simulink subsystem "gfmWind"  (R2025a)
settings: Solver=VariableStepAuto  StartTime=0.0  StopTime=10.0  RelTol=1e-3
model mask{Control=VSM Using DC Link Voltage, V_ref=V_ref, Q_ref=Q_ref, Kq=Kq_dc, Kt=Kt, KqI=Kq, Kp=Kp, Kd=Kd, Kj=Kj, H=H, D=D, Vd_ref=0, frequency1=0, frequency=0, Spref=Curtailed Power Operation, tstart=0, Vslope=0, Pstart=0, Pslope=0, x_vir=0, x_vir1=0, r_vir1=0, Imax1=0, Imax=0, r_vir=0, Kpq_mpp=Lq*alpha, Kpd_mpp=Ld*alpha, Kiq_mpp=Rs*alpha, Kid_mpp=Rs*alpha, Kpq=Lq*alpha, Kpd=Ld*alpha, Kiq=Rs*alpha, Kid=Rs*alpha, Kp_dc_sm=Kp_dc_sm, Ki_dc_sm=Ki_dc_sm, wt1=0, rt1=0, pitch1=0, cp1=0, airDensity1=0, TSR1=0, Radius1=0, wt=0.01, rt=0.01, pitch=pitch, cp=cp, airDensity=airDensity, Radius=turbineRadius, TSR=TSR, Inertia1=0, Inertia=0, psim1=0, p1=0, Rs1=0, Lq1=0, Ld1=0, Ld=Ld, Lq=Lq, Rs=Rs, p=p, psim=psim}
  mask prompts: Control "GFM Controller"; V_ref "Voltage Reference (PU)"; Q_ref "Reactive Power Reference"; Kq "Reactive Power Droop"; Kt "Tracking Coefficient"; KqI "VSM Reactive power droop"; Kp "VSM frequency droop"; Kd "Damping Coefficient"; Kj "Inertia Coefficient"; H "VSM Inertia"; D "VSM damping"; Vd_ref "Volatge Reference d-axis"; frequency1 "Frequency reference"; frequency "Reference frequency"; Spref "Select Real Power Rference (MW)"; tstart "Start time of Voltage ramp (s)"; Vslope "Slope of Voltage ramp (pu)"; Pstart "Start time of Power ramp (s)"; Pslope "Slope of Power ramp (pu)"; x_vir "Virtual reactance"; x_vir1 "Virtual reactance"; r_vir1 "Virtual resistance"; Imax1 "Current limit"; Imax "Current limit"; r_vir "Virtual resistance"; Kpq_mpp "Q-axis Proportional Gain"; Kpd_mpp "D-axis Proportional Gain"; Kiq_mpp "Q-axis Integral Gain"; Kid_mpp "D-axis Integral Gain"; Kpq "q-axis proportional Gain"; Kpd "D-axis proportional Gain"; Kiq "q-axis integral Gain"; Kid "D-axis integral Gain"; Kp_dc_sm "Prportional Gain of Dc-link Controller"; Ki_dc_sm "Integral Gain of DC-link Controller"; wt1 "Wind Velocity Threshold"; rt1 "Rotational Velocity Threshold"; pitch1 "Pitch Angle Vector"; cp1 "Power Coefficient Table"; airDensity1 "Air Density"; TSR1 "Tip Speed Ratio"; Radius1 "Radius of Turbine"; wt "Wind Velocity Threshold"; rt "Rotational Velocity Threshold"; pitch "Turbine Pitch Angle Vector"; cp "Power Coefficient"; airDensity "Air Density"; Radius "Turbine Radius"; TSR "Tip Speed Ratio"; Inertia1 "Turbine Inertia"; Inertia "Turbine Inertia"; psim1 "PM Flux Linkage"; p1 "Number of Pole Pairs"; Rs1 "Stator Resistance (Ohms)"; Lq1 "Stator Q-axis inductance (H)"; Ld1 "Stator D-axis inductance (H)"; Ld "Stator D-axis inductance (H)"; Lq "Stator Q-axis inductance (H)"; Rs "Stator Resistance (Ohms)"; p "Number of Pole Pairs"; psim "PMSM Flux linkage (Wb)"
settings Model: Creator=rajarshd  LastModifiedBy=rajarshd
settings RTWCC: GPUComputeCapability=3.5

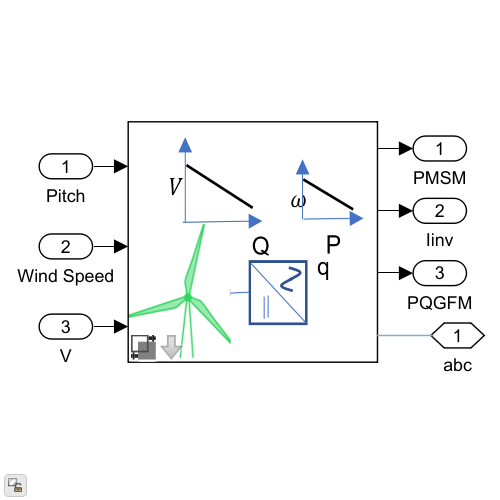
[thumbnail: Simulink's stored preview of the top-level diagram]
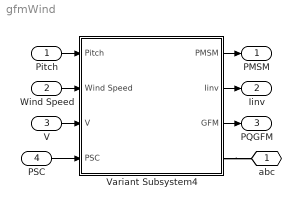
== system gfmWind ==
  Pitch : Inport
  Wind Speed : Inport  Port=2
  V : Inport  Port=3
  PSC : Inport  Port=4
  Variant Subsystem4 : Subsystem  Variant=on  VariantControlMode=label  LabelModeActiveChoice=WindVSMControlDClink  PropagateVariantConditions=on  mask{Control=VSM Using DC Link Voltage, KqI=KqI, Q_ref=Q_ref, Kp=Kp, H=H, D=D, V_ref=V_ref, Kq=Kq, Kt=Kt, Kj=Kj, Kd=Kd, Vd_ref=Vd_ref, frequency=frequency, frequency1=frequency1, Spref=Curtailed Power Operation, Pslope=Pslope, Pstart=Pstart, Vslope=Vslope, tstart=tstart, x_vir1=x_vir1, x_vir=x_vir, r_vir=r_vir, r_vir1=r_vir1, Imax=Imax, Imax1=Imax1, Kid=Kid, Kiq=Kiq, Kpd=Kpd, Kpq=Kpq, Ki_dc_sm=Ki_dc_sm, Kp_dc_sm=Kp_dc_sm, Kpq_mpp=Kpq_mpp, Kpd_mpp=Kpd_mpp, Kid_mpp=Kid_mpp, Kiq_mpp=Kiq_mpp, psim1=psim1, p1=p1, Rs1=Rs1, Lq1=Lq1, Ld1=Ld1, Ld=Ld, Lq=Lq, p=p, psim=psim, Rs=Rs, wt1=wt1, rt1=rt1, pitch1=pitch1, cp1=cp1, TSR1=TSR1, Radius1=Radius1, airDensity1=airDensity1, Radius=Radius, TSR=TSR, airDensity=airDensity, cp=cp, pitch=pitch, rt=rt, wt=wt, Inertia1=Inertia1, Inertia=Inertia}
      mask prompts: Control "GFM Controller"; KqI "VSM Reactive power droop"; Q_ref "Reactive Power Reference"; Kp "VSM frequency droop"; H "VSM Inertia"; D "VSM damping"; V_ref "Voltage Reference (PU)"; Kq "Reactive Power Droop"; Kt "Tracking Cofficient"; Kj "Inertia Cofficient"; Kd "Damping Cofficient"; Vd_ref "Volatge Reference d-axis"; frequency "Reference frequency"; frequency1 "Frequency reference"; Spref "Select Real Power Rference (MW)"; Pslope "Slope of Power ramp (pu)"; Pstart "Start time of Power ramp (s)"; Vslope "Slope of Voltage ramp (pu)"; tstart "Start time of Voltage ramp (s)"; x_vir1 "Virtual reactance"; x_vir "Virtual reactance"; r_vir "Virtual resistance"; r_vir1 "Virtual resistance"; Imax "Current limit"; Imax1 "Current limit"; Kid "D-axis integral Gain"; Kiq "q-axis integral Gain"; Kpd "D-axis proportional Gain"; Kpq "q-axis proportional Gain"; Ki_dc_sm "Integral Gain of DC-link Controller"; Kp_dc_sm "Prportional Gain of Dc-link Controller"; Kpq_mpp "Q-axis Proportional Gain"; Kpd_mpp "D-axis Proportional Gain"; Kid_mpp "D-axis Integral Gain"; Kiq_mpp "Q-axis Integral Gain"; psim1 "PM Flux Linkage"; p1 "Number of Pole Pairs"; Rs1 "Stator Resistance (Ohms)"; Lq1 "Stator Q-axis inductance (H)"; Ld1 "Stator D-axis inductance (H)"; Ld "Stator D-axis inductance (H)"; Lq "Stator Q-axis inductance (H)"; p "Number of Pole Pairs"; psim "PMSM Flux linkage (Wb)"; Rs "Stator Resistance (Ohms)"; wt1 "Wind Velocity Threshold"; rt1 "Rotational Velocity Threshold"; pitch1 "Pitch Angle Vector"; cp1 "Power Cofficient Table"; TSR1 "Tip Speed Ratio"; Radius1 "Radious of Turbine"; airDensity1 "Air Density"; Radius "Turbine Radious"; TSR "Tip Speed Ratio"; airDensity "Air Density"; cp "Power Cofficient"; pitch "Turbine Pitch Angle Vector"; rt "Rotational Velocity Threshold"; wt "Wind Velocity Threshold"; Inertia1 "Turbine Inertia"; Inertia "Turbine Inertia"
      mask init:
      | Choice = get_param(gcb,'Control');
      | switch Choice
      |     case 'VSM Using DC Link Voltage'
      |         set_param(gcb, 'LabelModeActiveChoice', 'WindVSMControlDClink')
      |     case 'VSM Using Turbine Inertia'
      |          set_param(gcb, 'LabelModeActiveChoice', 'WindVSMControlTurbineInertia')
      |    otherwise
      |         disp('Choose proper active power control method')
      | end
      mask TypeOptions Control: VSM Using Turbine Inertia | VSM Using DC Link Voltage
      mask Callback Control:
      | h = Simulink.Mask.get(gcb);
      | Choice = get_param(gcb,'Control');
      | switch Choice
      |     case 'VSM Using DC Link Voltage'
      |         set_param(gcb, 'LabelModeActiveChoice', 'WindVSMControlDClink')
      |     case 'VSM Using Turbine Inertia'
      |          set_param(gcb, 'LabelModeActiveChoice', 'WindVSMControlTurbineInertia')
      | end
      mask TypeOptions KqI: VSM Inertia/KqI
      mask TypeOptions Q_ref: VSM DC/Q_ref
      mask TypeOptions Kp: VSM Inertia/Kp
      mask TypeOptions H: VSM Inertia/H
      mask TypeOptions D: VSM Inertia/D
      mask TypeOptions V_ref: VSM DC/V_ref
      mask TypeOptions Kq: VSM DC/Kq
      mask TypeOptions Kt: VSM DC/Kt
      mask TypeOptions Kj: VSM DC/Kj
      mask TypeOptions Kd: VSM DC/Kd
      mask TypeOptions Vd_ref: VSM Inertia/Vd_ref
      mask TypeOptions frequency: VSM Inertia/frequency
      mask TypeOptions frequency1: VSM DC/frequency1
      mask TypeOptions Spref: VSM Inertia/Spref
      mask TypeOptions Pslope: VSM Inertia/Pslope
      mask TypeOptions Pstart: VSM Inertia/Pstart
      mask TypeOptions Vslope: VSM Inertia/Vslope
      mask TypeOptions tstart: VSM Inertia/tstart
      mask TypeOptions x_vir1: VSM DC/x_vir1
      mask TypeOptions x_vir: VSM Inertia/x_vir
      mask TypeOptions r_vir: VSM Inertia/r_vir
      mask TypeOptions r_vir1: VSM DC/r_vir1
      mask TypeOptions Imax: VSM Inertia/Imax
      mask TypeOptions Imax1: VSM DC/Imax1
      mask TypeOptions Kid: VSM Inertia/Kid
      mask TypeOptions Kiq: VSM Inertia/Kiq
      mask TypeOptions Kpd: VSM Inertia/Kpd
      mask TypeOptions Kpq: VSM Inertia/Kpq
      mask TypeOptions Ki_dc_sm: VSM Inertia/Ki_dc_sm
      mask TypeOptions Kp_dc_sm: VSM Inertia/Kp_dc_sm
      mask TypeOptions Kpq_mpp: VSM DC/Kpq_mpp
      mask TypeOptions Kpd_mpp: VSM DC/Kpd_mpp
      mask TypeOptions Kid_mpp: VSM DC/Kid_mpp
      mask TypeOptions Kiq_mpp: VSM DC/Kiq_mpp
      mask TypeOptions psim1: VSM Inertia/psim1
      mask TypeOptions p1: VSM Inertia/p1
      mask TypeOptions Rs1: VSM Inertia/Rs1
      mask TypeOptions Lq1: VSM Inertia/Lq1
      mask TypeOptions Ld1: VSM Inertia/Ld1
      mask TypeOptions Ld: VSM DC/Ld
      mask TypeOptions Lq: VSM DC/Lq
      mask TypeOptions p: VSM DC/p
      mask TypeOptions psim: VSM DC/psim
      mask TypeOptions Rs: VSM DC/Rs
      mask TypeOptions wt1: VSM Inertia/wt1
      mask TypeOptions rt1: VSM Inertia/rt1
      mask TypeOptions pitch1: VSM Inertia/pitch1
      mask TypeOptions cp1: VSM Inertia/cp1
      mask TypeOptions TSR1: VSM Inertia/TSR1
      mask TypeOptions Radius1: VSM Inertia/Radius1
      mask TypeOptions airDensity1: VSM Inertia/airDensity1
      mask TypeOptions Radius: VSM DC/Radius
      mask TypeOptions TSR: VSM DC/TSR
      mask TypeOptions airDensity: VSM DC/airDensity
      mask TypeOptions cp: VSM DC/cp
      mask TypeOptions pitch: VSM DC/pitch
      mask TypeOptions rt: VSM DC/rt
      mask TypeOptions wt: VSM DC/wt
      mask TypeOptions Inertia1: VSM Inertia/Inertia1
      mask TypeOptions Inertia: VSM DC/Inertia
      mask DialogControl Container4 Prompt: VSM Parameters
      mask DialogControl Container8 Prompt: Fault Ridethrough Parameters
      mask DialogControl Container5 Prompt: PMSM Controller
      mask DialogControl Container6 Prompt: PMSM Parameters
      mask DialogControl Container7 Prompt: Wind Turbine Parameters
      mask Display: image('WindGFM.png')
  abc : PMIOPort  Side=Right
  PMSM : Outport
  Iinv : Outport  Port=2
  PQGFM : Outport  Port=3
  wires:
  Variant Subsystem4/3(GFM) -> PQGFM/1
  Wind Speed/1 -> Variant Subsystem4/2(Wind Speed)
  V/1 -> Variant Subsystem4/3(V)
  Variant Subsystem4/1(PMSM) -> PMSM/1
  Pitch/1 -> Variant Subsystem4/1(Pitch)
  Variant Subsystem4/2(Iinv) -> Iinv/1
  PSC/1 -> Variant Subsystem4/4(PSC)
  connections:
  Variant Subsystem4/RConn1 -- abc/RConn1

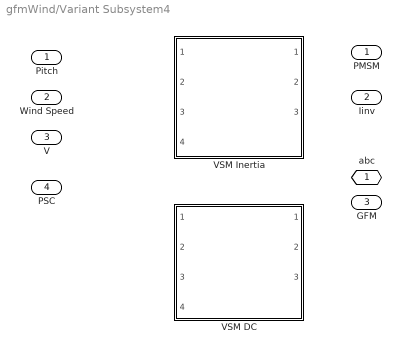
== system gfmWind/Variant Subsystem4 ==
  Pitch : Inport
  Wind Speed : Inport  Port=2
  V : Inport  Port=3
  PSC : Inport  Port=4
  VSM DC : Subsystem  VariantControl=WindVSMControlDClink  ReferencedSubsystem=WindGFMCap  x_vir1=x_vir1  r_vir1=r_vir1  Imax1=Imax1  Kt=Kt  Kj=Kj  Kd=Kd  frequency1=frequency1  V_ref=V_ref  Kq=Kq  Q_ref=Q_ref  Kpd_mpp=Kpd_mpp  Kid_mpp=Kid_mpp  Kpq_mpp=Kpq_mpp  Kiq_mpp=Kiq_mpp  p=p  psim=psim  Ld=Ld  Lq=Lq  Rs=Rs  Radius=Radius  pitch=pitch  cp=cp  TSR=TSR  airDensity=airDensity  wt=wt  rt=rt  Inertia=Inertia
  VSM Inertia : Subsystem  VariantControl=WindVSMControlTurbineInertia  ReferencedSubsystem=WindGFMTurbineInertia  Kp=Kp  D=D  H=H  KqI=KqI  Vd_ref=Vd_ref  frequency=frequency  Spref=Curtailed Power Operation  tstart=tstart  Vslope=Vslope  Pstart=Pstart  Pslope=Pslope  x_vir=x_vir  r_vir=r_vir  Imax=Imax  Radius1=Radius1  pitch1=pitch1  cp1=cp1  TSR1=TSR1  airDensity1=airDensity1  wt1=wt1  rt1=rt1  Inertia1=Inertia1  p1=p1  psim1=psim1  Ld1=Ld1  Lq1=Lq1  Rs1=Rs1  Kp_dc_sm=Kp_dc_sm  Ki_dc_sm=Ki_dc_sm  Kpd=Kpd  Kid=Kid  Kpq=Kpq  Kiq=Kiq
  abc : PMIOPort  Side=Right
  PMSM : Outport
  Iinv : Outport  Port=2
  GFM : Outport  Port=3
